simulink model "Simulink_progetto_non_linearizzato"  (R2023b)
settings: Solver=VariableStepAuto  StartTime=0.0  StopTime=0.02  RelTol=1e-3
values from neighbouring files (symbols this model uses):
  C_e = [1,0]    [ProgettoB2.m]
  u_e = k*x1_e    (= 65.4498469498)    [ProgettoB2.m]
  x_e = [x1_e; x2_e]    [ProgettoB2.m]
libraries: cstblocks x1
settings Model: Creator=guidocarnevale  LastModifiedBy=aleor

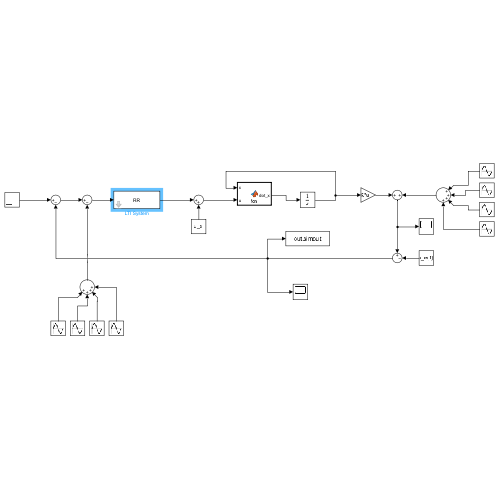
[thumbnail: Simulink's stored preview of the top-level diagram]
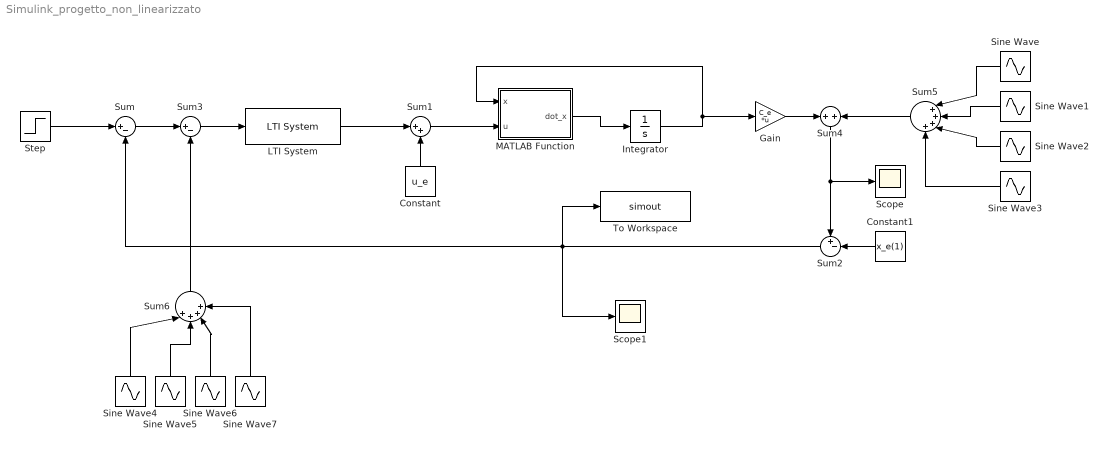
== system Simulink_progetto_non_linearizzato ==
  Constant : Constant  Value=u_e
  Constant1 : Constant  Value=x_e(1)
  Gain : Gain  Gain=C_e  Multiplication=Matrix(K*u)
  Integrator : Integrator  InitialCondition=x_e
  LTI System : cstblocks/LTI System  Tag=R  sys=RR  IC=[]  PadeOrder=0
  MATLAB Function : MATLAB Function  TreatAsAtomicUnit=on
  Scope : Scope
  Scope1 : Scope
  Sine Wave : Sin  Amplitude=10  Frequency=0.15  SampleTime=0
  Sine Wave1 : Sin  Amplitude=10  Frequency=0.30  SampleTime=0
  Sine Wave2 : Sin  Amplitude=10  Frequency=0.45  SampleTime=0
  Sine Wave3 : Sin  Amplitude=10  Frequency=0.60  SampleTime=0
  Sine Wave4 : Sin  Frequency=100000  SampleTime=0
  Sine Wave5 : Sin  Frequency=200000  SampleTime=0
  Sine Wave6 : Sin  Frequency=300000  SampleTime=0
  Sine Wave7 : Sin  Frequency=400000  SampleTime=0
  Step : Step  Time=0  SampleTime=0
  Sum : Sum  Inputs=|+-
  Sum1 : Sum  Inputs=|++
  Sum2 : Sum  Inputs=+-|
  Sum3 : Sum  Inputs=|+-
  Sum4 : Sum  Inputs=+|+
  Sum5 : Sum  Inputs=|++++
  Sum6 : Sum  Inputs=|++++
  To Workspace : ToWorkspace  VariableName=simout  SaveFormat=Timeseries  SampleTime=-1
  wires:
  MATLAB Function/1(dot_x) -> Integrator/1
  Integrator/1 -> MATLAB Function/1(x), Gain/1
  Sum/1 -> Sum3/1
  LTI System/1 -> Sum1/1
  Constant/1 -> Sum1/2
  Sum1/1 -> MATLAB Function/2(u)
  Sum3/1 -> LTI System/1
  Gain/1 -> Sum4/1
  Sum4/1 -> Scope/1, Sum2/1
  Constant1/1 -> Sum2/2
  Sum2/1 -> To Workspace/1, Scope1/1, Sum/2
  Step/1 -> Sum/1
  Sum5/1 -> Sum4/2
  Sum6/1 -> Sum3/2
  Sine Wave/1 -> Sum5/1
  Sine Wave2/1 -> Sum5/3
  Sine Wave1/1 -> Sum5/2
  Sine Wave3/1 -> Sum5/4
  Sine Wave7/1 -> Sum6/4
  Sine Wave6/1 -> Sum6/3
  Sine Wave4/1 -> Sum6/1
  Sine Wave5/1 -> Sum6/2

== matlab function Simulink_progetto_non_linearizzato/MATLAB Function ==
  data: x input; u input; dot_x output
function dot_x = fcn(x,u)
% Coefficienti momento d'inerzia
J_0=8;
J_1=0.4;
J_2=0.4;
J_3=0.5;
J_4=0.7;

psi_1=-0.1;
psi_2=2;
psi_3=2.5;
psi_4=-1;

% Momento d'inerzia
J = @(x) J_0 + J_1 * cos(x + psi_1)+ J_2 * cos(2*x + psi_2)+ J_3 * cos(3*x + psi_3)+ J_4 * cos(4*x + psi_4);

beta=15;
k = 50;

dot_x = zeros(2,1);

dot_x(1) = x(2);

dot_x(2) = (u-beta*x(2)-k*x(1))/J(x(1));
